simulink model "sm_stewart_platform"  (R2019b)
settings: Solver=ode45  StartTime=0.0  StopTime=450  MaxStep=0.2  RelTol=1e-3  EnableMultiTasking=on
model workspace (MAT data in the model file):
  g_density = 5
values from neighbouring files (symbols this model uses):
  B = base_points.Data(:,:,1)    [run_this_for_sim.m]
  base_radius = 0.75*100    (= 75)    [run_this_for_sim.m]
  desired_max_angle = 10    [run_this_for_sim.m]
  desired_max_x = 0.05    [run_this_for_sim.m]
  desired_max_y = desired_max_x    (= 0.05)    [run_this_for_sim.m]
  desired_max_z = 0.05    [run_this_for_sim.m]
  initial_integral_force = 200    [run_this_for_sim.m]
  leg_max = leg_min+0.3    (= 1.322)    [run_this_for_sim.m]
  leg_min = 1.022    [run_this_for_sim.m]
  leg_thickness = 75/1000    (= 0.075)    [run_this_for_sim.m]
  lower_leg_length = upper_leg_length    (= 0.511)    [run_this_for_sim.m]
  max_velocity = 0.15    [run_this_for_sim.m]
  P = platform_points.Data(:,:,1)    [run_this_for_sim.m]
  platform_radius = 0.75*base_radius    (= 56.25)    [run_this_for_sim.m]
  platform_thickness = 0.1/8    (= 0.0125)    [run_this_for_sim.m]
  trajectory_smoothing = 1/1.5    (= 0.666666666667)    [run_this_for_sim.m]
  upper_leg_length = dead_length/2    (= 0.511)    [run_this_for_sim.m]
  work_height = 1.2*100    (= 120)    [run_this_for_sim.m]
undefined symbols (not defined in the file or in its folder): nom_length, X, Z
libraries: sp_lib x18, nesl_utility x11, sm_lib x9, simulink x2
(part 2 of 10)

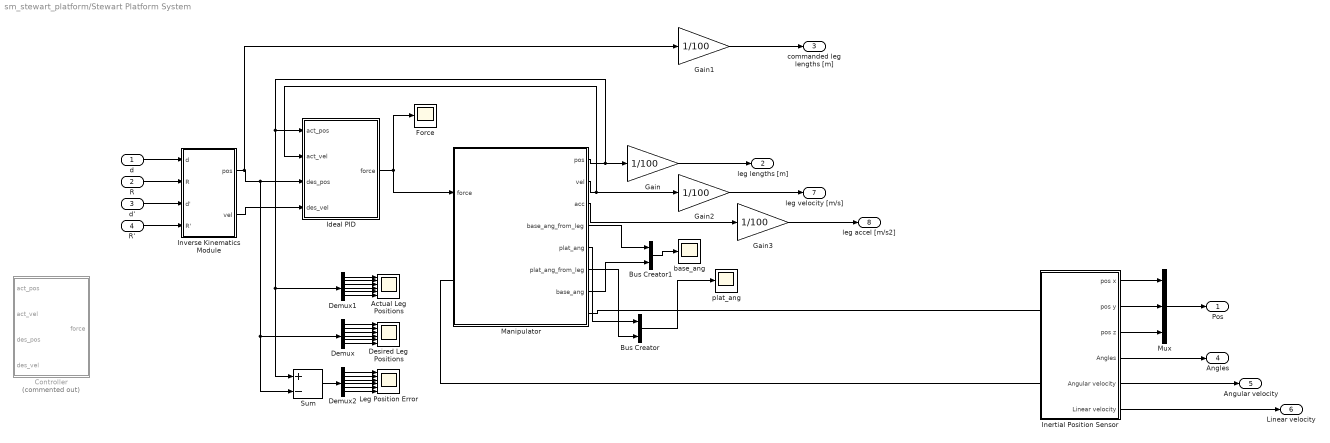
== system sm_stewart_platform/Stewart Platform System ==
  d : Inport
  R : Inport  Port=2
  d' : Inport  Port=3
  R' : Inport  Port=4
  Actual Leg Positions : Scope  NumInputPorts=6
  Bus Creator : BusCreator  Inputs=2
  Bus Creator1 : BusCreator  Inputs=2
  Controller : Subsystem  Commented=on  mask(PID Controller){Kp=Kp, Ki=Ki, Kd=Kd}
      mask prompts: Kp "Proportional Gain"; Ki "Integral Gain"; Kd "Derivative Gain"
      mask help:
      | Generates an actuation output based on a desired trajectory and an actual trajectory, using a generic proportional-integral-derivative (PID) control law.  The three control gains are specified through parameters.
      |
      | Both the desired and actual trajectories are specified by separate position and velocity input signals.  The controller is generic and can control to trajectories through state spaces of arbitrary dimension; the only requirement is that all four inputs have the same dimension.
      mask Help:
      | A <em>PID Controller</em> generates an actuation output based on a desired trajectory and an actual trajectory, using a generic proportional-integral-derivative (PID) control law.  The three control gains are specified through parameters.
      | 
      | Both the desired and actual trajectories are specified by separate position and velocity input signals.  The controller is generic and can control to trajectories through state spaces of arbitrary dimension; the only requirement is that all four inputs have the same dimension.
      | 
      | This block is not specific to the Stewart platform and could serve in any general purpose control library.  For the Stewart platform application, the trajectories are all through the 6-D leg-position space.
      | 
      | <h3>Gains</h3>
      | 
      | The parameters specify the gains of the controller.
      | 
      | <ul>
      | 
      | <li> <b>Proportional Gain</b> The gain that determines the strength of the control actuation in response to current deviations between actual and desired positions.  This affects the responsiveness of the controller but can lead to instability if set too high.
      | 
      | <li> <b>Integral Gain</b> The gain that determines the strength of the control actuation in response to deviations between actual and desired positions that persist over time.  A nonzero integral term is often necessary to avoid <em>droop</em> (steady-state error).  Higher values reduce the transient response of the controller but can cause overshoot in the controlled position.
      | 
      | <li> <b>Derivative Gain</b> The gain that determines the strength of the control actuation in response to the derivative of the deviations between actual and desired positions.  This is a damping component used to reduce overshoot in the controlled position; the tradeoff is that it reduces the transient response of the controller.  Higher values increase the stiffness of the system and can lead to instability.
      | 
      | </ul>
      | 
      | 
      | <h3>Ports</h3>
      | 
      | <ul>
      | 
      | <li> <b>act_pos</b> The current actual position of the plant.
      | 
      | <li> <b>act_pos</b> The current actual velocity of the plant.  This should be the time derivative of the <em>act_pos</em> signal.
      | 
      | <li> <b>des_pos</b> The current desired position of the plant.
      | 
      | <li> <b>des_pos</b> The current desired velocity of the plant.  This should be the time derivative of the <em>des_pos</em> signal.
      | 
      | </ul>
  Demux : Demux  Outputs=6
  Demux1 : Demux  Outputs=6
  Demux2 : Demux  Outputs=6
  Desired Leg Positions : Scope  NumInputPorts=6
  Force : Scope
  Gain{,1..3} (4 alike) : Gain  Gain=1/100
  Ideal PID : Subsystem  mask(PID Controller){Kp=Kp, Ki=Ki, Kd=Kd}
      mask prompts: Kp "Proportional Gain"; Ki "Integral Gain"; Kd "Derivative Gain"
      mask help:
      | Generates an actuation output based on a desired trajectory and an actual trajectory, using a generic proportional-integral-derivative (PID) control law.  The three control gains are specified through parameters.
      |
      | Both the desired and actual trajectories are specified by separate position and velocity input signals.  The controller is generic and can control to trajectories through state spaces of arbitrary dimension; the only requirement is that all four inputs have the same dimension.
      mask Help:
      | A <em>PID Controller</em> generates an actuation output based on a desired trajectory and an actual trajectory, using a generic proportional-integral-derivative (PID) control law.  The three control gains are specified through parameters.
      | 
      | Both the desired and actual trajectories are specified by separate position and velocity input signals.  The controller is generic and can control to trajectories through state spaces of arbitrary dimension; the only requirement is that all four inputs have the same dimension.
      | 
      | This block is not specific to the Stewart platform and could serve in any general purpose control library.  For the Stewart platform application, the trajectories are all through the 6-D leg-position space.
      | 
      | <h3>Gains</h3>
      | 
      | The parameters specify the gains of the controller.
      | 
      | <ul>
      | 
      | <li> <b>Proportional Gain</b> The gain that determines the strength of the control actuation in response to current deviations between actual and desired positions.  This affects the responsiveness of the controller but can lead to instability if set too high.
      | 
      | <li> <b>Integral Gain</b> The gain that determines the strength of the control actuation in response to deviations between actual and desired positions that persist over time.  A nonzero integral term is often necessary to avoid <em>droop</em> (steady-state error).  Higher values reduce the transient response of the controller but can cause overshoot in the controlled position.
      | 
      | <li> <b>Derivative Gain</b> The gain that determines the strength of the control actuation in response to the derivative of the deviations between actual and desired positions.  This is a damping component used to reduce overshoot in the controlled position; the tradeoff is that it reduces the transient response of the controller.  Higher values increase the stiffness of the system and can lead to instability.
      | 
      | </ul>
      | 
      | 
      | <h3>Ports</h3>
      | 
      | <ul>
      | 
      | <li> <b>act_pos</b> The current actual position of the plant.
      | 
      | <li> <b>act_pos</b> The current actual velocity of the plant.  This should be the time derivative of the <em>act_pos</em> signal.
      | 
      | <li> <b>des_pos</b> The current desired position of the plant.
      | 
      | <li> <b>des_pos</b> The current desired velocity of the plant.  This should be the time derivative of the <em>des_pos</em> signal.
      | 
      | </ul>
  Inertial Position Sensor : Subsystem
  Inverse Kinematics Module : Subsystem  mask(Stewart Platform Inverse Kinematics){}
      mask help:
      | Performs the essential inverse kinematic computations for a Stewart platform manipulator.
      |
      | Given a desired dynamic state of a Stewart platform manipulator specified by a 3-D rigid transformation from the gripper frame to the base reference frame, and the first time derivative of this transformation, this block computes the positions and velocities of the prismatic primitives of the six cylindrical leg joints necessary to achieve the desired dynamic state.
      mask Help:
      | A <em>Stewart Platform Inverse Kinematics</em> performs the essential inverse kinematic computations for a Stewart platform manipulator.
      | 
      | Given a desired dynamic state of a Stewart platform manipulator specified by a 3-D rigid transformation from the gripper frame to the base reference frame, and the first time derivative of this transformation, this block computes the positions and velocities of the prismatic primitives of the six cylindrical leg joints necessary to achieve the desired dynamic state.
      | 
      | <h3>Manipulator Transformation</h3>
      | 
      | The desired dynamic state of a Stewart platform manipulator may be specified by a single 3-D rigid transformation, called the <em>manipulator transformation</em>, and its time derivative.  The transformation is from <em>gripper</em> frame to <em>base</em> frame coordinates.  The base frame is attached to the base plate of the manipulator.  Its origin is located at the center of the base, and the z-axis points directly upward.  The gripper frame is located somewhere directly above the center of platform plate of the manipulator, and is aligned with the base frame when the positions of the prismatic primitives of all six cylindrical leg joints are equal.
      | 
      | In the following discussions, let <b>R</b> and <b>d</b> specify the rotation matrix and displacement vector, respectively, of the manipulator transformation. That is, <b>d</b> is the origin of the gripper frame specified in base frame coordinates, and the columns of <b>R</b> are the canonical <b>i</b>, <b>j</b>, and <b>k</b> vectors of the gripper frame resolved in base frame coordinates.
      | Let <b>R'</b> and <b>d'</b> be the first time derivatives of <b>R</b> and <b>d</b>, respectively.
      | 
      | <h3>Inverse Kinematics</h3>
      | 
      | Each of the six legs of the manipulator is attached between a pair of universal joints: one on the base plate and one on the platform plate.  Each leg has an internal knee joint with a sensed and actuated prismatic primitive.
      | Let <em>q_i</em> and <em>q_i'</em> be the position and velocity of this primitive on Leg <em>i</em>.  Let <em>L0</em> denote the <em>nominal</em> lengths of the legs.  This is the length of a leg when its prismatic primitive is at the zero position.
      | 
      | The goal of the inverse kinematics computation is to determine the values of <em>q_i</em> and <em>q_i'</em> for i = 1, ..., 6 needed to achieve a particular manipulator transformation and its derivative.
      | 
      | The key to understanding the inverse kinematics computations is to consider the positions of the centers of the pairs of universal joints.  (These points are the centers of the crosspieces visible in the visualization of the manipulator.)
      | 
      | Let <b>b</b>_i and <b>p</b>_i be the 3-D points specifying the center of the universal joints on the base and platform plates, respectively, to which Leg <em>i</em> is connected. <b>b</b>_i is specified in base frame coordinates, and <b>p</b>_i is specified in gripper frame coordinates.  Then the desired position of the prismatic primitive of the knee joint of Leg <em>i</em> is given by
      | 
      | <em>q_i</em> = || <b>R</b> <b>p</b>_i + <b>d</b> - <b>b</b>_i || - <em>L0</em>.
      | 
      | Denote the vector within the norm expression above as <b>o</b>_i (<b>o</b> for <em>offset</em>).
      | 
      | The desired velocity of the prismatic primitive of the knee joint of Leg <em>i</em> is obtained by differentiating the expression for <em>q_i</em>. Noting that <b>p</b>_i, <b>b</b>_i, and <em>L0</em> are constant, the result is:
      | 
      | <em>q_i'</em> = [ (<b>R'</b> <b>p</b>_i + <b>d'</b>) . <b>o</b>_i ] / || <b>o</b>_i ||.
      | 
      | Note that the denominator of this expression is equal to the vector norm in the expression for <em>q_i</em>.
      | 
      | This block computes the values of all six prismatic primitive positions and velocities according to the expressions above.  The computation of the (constant) <b>p</b>_i and <b>b</b>_i points is highly dependent on the manipulator kinematics and done in the mask initialization of the containing <em>Stewart Platform System</em> block.
      | 
      | <h3>Ports</h3>
      | 
      | <ul>
      | 
      | <li> <b>d</b> The displacement vector of the desired manipulator transformation (see above) in units of centimeters.
      | 
      | <li> <b>R</b> The rotation matrix of the desired manipulator transformation (see above).
      | 
      | <li> <b>d'</b> The time derivative of the displacement vector of the desired manipulator transformation in units of centimeters/second.
      | 
      | <li> <b>R'</b> The time derivative of the rotation matrix of the desired manipulator transformation.
      | 
      | <li> <b>pos</b> The computed positions of the prismatic primitives of the six leg joints, as a 6 x 1 vector in units of centimeters.
      | 
      | <li> <b>vel</b> The computed velocities of the prismatic primitives of the six leg joints, as a 6 x 1 vector in units of centimeters/second.
      | 
      | 
      | </ul>
      | 
      | <!--  LocalWords:  ith pos vel
      |  -->
  Leg Position Error : Scope  NumInputPorts=6
  Manipulator : Subsystem  mask(Stewart Platform Manipulator){}
      mask help: Models the mechanical portion of a complete Stewart platform manipulator system: the manipulator itself. Almost all of the Simscape Multibody blocks of the full system are contained in the manipulator subsystem.
      mask Help:
      | A <em>Stewart Platform Manipulator</em> models the mechanical portion of a complete Stewart platform manipulator system: the manipulator itself.  Almost all of the Simscape Multibody blocks of the full system are contained in the manipulator subsystem.
      | 
      | The manipulator subsystem exposes two frames: the world frame, to which the base is anchored, and the gripper frame, which is the frame at the distil end of the end effector.  Typically, a user wants to control the manipulator transformation, which is the 3-D rigid transformation from the gripper frame to the world frame.
      | 
      | The manipulator subsystem has no internal control.  However, it reports the positions and velocities of the prismatic primitives of all six cylindrical leg joints as output signals and takes the actuation forces to be applied to these primitives as input signals.  When connected to an appropriate controller, these signals are sufficient to provide any of a variety of control schemes for the manipulator.
      | 
      | <h3>Parameterization</h3>
      | 
      | The manipulator is highly parameterized.  Most of the physical dimensions of its component pieces can be controlled via parameters.  These parameters are all defined in the containing <em>Stewart Platform System</em>.  The manipulator's parameters are inherited from that block; they are not defined explicitly in this block's mask.  The parameters are also needed for the <em>Stewart Platform Inverse Kinematics</em> block.
      | 
      | See the documentation of the <em>Stewart Platform System</em> block for details.
      | 
      | <h3>Ports</h3>
      | 
      | <ul>
      | 
      | <li> <b>gripper</b> The gripper frame.  This frame is fixed at the distil end of the end effector attached to the platform plate of the Stewart platform manipulator.  It is identified with a frame glyph in the visualization of the manipulator.  Typically, a user of the manipulator wants to control the pose of this frame, with respect to a reference frame such as world.
      | 
      | <li> <b>world</b> The world frame.  This is also the reference frame of the base plate of the Stewart platform manipulator, which is rigidly attached to the world frame.
      | 
      | <li><b>pos</b> The positions of the prismatic primitives of the six leg joints as a 6 x 1 output signal in units of centimeters.
      | 
      | <li><b>vel</b> The velocities of the prismatic primitives of the six leg joints as a 6 x 1 output signal in units of centimeters/second.
      | 
      | <li><b>force</b> The actuation forces applied to the prismatic primitives of the six leg joints as a 6 x 1 input signal in units of Newtons.
      | 
      | </ul>
      | 
      | <!--  LocalWords:  Eff IC Ctrl pos vel
      |  -->
      mask Display:
      | image(imread('sm_stewart_platform_manipulator.png'))
      | color('white')
      | port_label('LConn', 1, 'world')
      | port_label('RConn', 1, 'gripper')
      | color('yellow')
      | port_label('Input', 1, 'force')
      | port_label('Output', 1, 'pos')
      | port_label('Output', 2, 'vel')
      | port_label('Output', 3, 'acc')
      | port_label('Output', 4, 'base_ang')
      | port_label('Output', 5, 'plat_ang')
  Mux : Mux  Inputs=3
  Sum : Sum  Inputs=+-
  base_ang : Scope
  plat_ang : Scope
  Pos : Outport  VectorParamsAs1DForOutWhenUnconnected=off
  leg lengths [m] : Outport  Port=2  VectorParamsAs1DForOutWhenUnconnected=off
  commanded leg lengths [m] : Outport  Port=3  VectorParamsAs1DForOutWhenUnconnected=off
  Angles : Outport  Port=4  VectorParamsAs1DForOutWhenUnconnected=off
  Angular velocity : Outport  Port=5  VectorParamsAs1DForOutWhenUnconnected=off
  Linear velocity : Outport  Port=6  VectorParamsAs1DForOutWhenUnconnected=off
  leg velocity [m/s] : Outport  Port=7  VectorParamsAs1DForOutWhenUnconnected=off
  leg accel [m/s2] : Outport  Port=8  VectorParamsAs1DForOutWhenUnconnected=off
  wires:
  Manipulator/2(vel) -> Ideal PID/2(act_vel), Gain2/1
  d/1 -> Inverse Kinematics Module/1(d)
  R/1 -> Inverse Kinematics Module/2(R)
  Demux/1 -> Desired Leg Positions/1
  Demux/2 -> Desired Leg Positions/2
  Demux/3 -> Desired Leg Positions/3
  Demux/4 -> Desired Leg Positions/4
  Demux/5 -> Desired Leg Positions/5
  Demux/6 -> Desired Leg Positions/6
  Demux1/1 -> Actual Leg Positions/1
  Demux1/2 -> Actual Leg Positions/2
  Demux1/3 -> Actual Leg Positions/3
  Demux1/4 -> Actual Leg Positions/4
  Demux1/5 -> Actual Leg Positions/5
  Demux1/6 -> Actual Leg Positions/6
  Demux2/1 -> Leg Position Error/1
  Demux2/2 -> Leg Position Error/2
  Demux2/3 -> Leg Position Error/3
  Demux2/4 -> Leg Position Error/4
  Demux2/5 -> Leg Position Error/5
  Demux2/6 -> Leg Position Error/6
  Sum/1 -> Demux2/1
  d'/1 -> Inverse Kinematics Module/3(d')
  R'/1 -> Inverse Kinematics Module/4(R')
  Ideal PID/1(force) -> Force/1, Manipulator/1(force)
  Manipulator/1(pos) -> Ideal PID/1(act_pos), Demux1/1, Sum/1, Gain/1
  Inertial Position Sensor/1(pos x) -> Mux/1
  Inertial Position Sensor/2(pos y) -> Mux/2
  Inertial Position Sensor/3(pos z) -> Mux/3
  Mux/1 -> Pos/1
  Inverse Kinematics Module/2(vel) -> Ideal PID/4(des_vel)
  Inverse Kinematics Module/1(pos) -> Gain1/1, Ideal PID/3(des_pos), Sum/2, Demux/1
  Gain/1 -> leg lengths [m]/1
  Gain1/1 -> commanded leg lengths [m]/1
  Inertial Position Sensor/4(Angles) -> Angles/1
  Inertial Position Sensor/5(Angular velocity) -> Angular velocity/1
  Inertial Position Sensor/6(Linear velocity) -> Linear velocity/1
  Gain2/1 -> leg velocity [m/s]/1
  Gain3/1 -> leg accel [m/s2]/1
  Manipulator/3(acc) -> Gain3/1
  Manipulator/5(plat_ang) -> Bus Creator/1
  Bus Creator/1 -> plat_ang/1
  Manipulator/6(plat_ang_from_leg) -> Bus Creator/2
  Manipulator/4(base_ang_from_leg) -> Bus Creator1/1
  Manipulator/7(base_ang) -> Bus Creator1/2
  Bus Creator1/1 -> base_ang/1
  connections:
  Inertial Position Sensor/LConn1 -- Manipulator/RConn1
  Inertial Position Sensor/LConn2 -- Manipulator/LConn1
